simulink model "TST_EGRVlv_VDMon"  (R2016b)
settings: Solver=FixedStepDiscrete  StartTime=0.0  StopTime=simTime  FixedStep=sampleTime  RelTol=1e-3
values from neighbouring files (symbols this model uses):
  testCase = 1    [initTST_EGRVlv_VDMon_001.m]
libraries: UnitTest_Lib x6, simulink x2
settings Model: Creator=liangyunbo  LastModifiedBy=liangyunbo
settings DebuggingCC: SignalRangeChecking=error

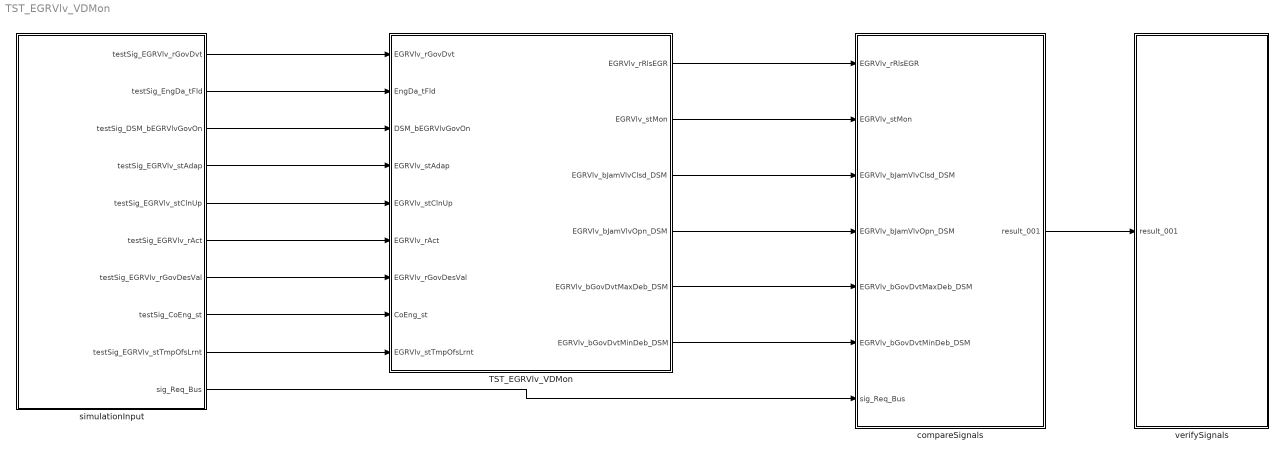
== system TST_EGRVlv_VDMon ==
  TST_EGRVlv_VDMon : Subsystem
  compareSignals : Subsystem
  simulationInput : Subsystem
  verifySignals : Subsystem
  wires:
  simulationInput/1(testSig_EGRVlv_rGovDvt) -> TST_EGRVlv_VDMon/1(EGRVlv_rGovDvt)
  simulationInput/2(testSig_EngDa_tFld) -> TST_EGRVlv_VDMon/2(EngDa_tFld)
  simulationInput/3(testSig_DSM_bEGRVlvGovOn) -> TST_EGRVlv_VDMon/3(DSM_bEGRVlvGovOn)
  simulationInput/4(testSig_EGRVlv_stAdap) -> TST_EGRVlv_VDMon/4(EGRVlv_stAdap)
  simulationInput/5(testSig_EGRVlv_stClnUp) -> TST_EGRVlv_VDMon/5(EGRVlv_stClnUp)
  simulationInput/6(testSig_EGRVlv_rAct) -> TST_EGRVlv_VDMon/6(EGRVlv_rAct)
  simulationInput/7(testSig_EGRVlv_rGovDesVal) -> TST_EGRVlv_VDMon/7(EGRVlv_rGovDesVal)
  simulationInput/8(testSig_CoEng_st) -> TST_EGRVlv_VDMon/8(CoEng_st)
  simulationInput/9(testSig_EGRVlv_stTmpOfsLrnt) -> TST_EGRVlv_VDMon/9(EGRVlv_stTmpOfsLrnt)
  TST_EGRVlv_VDMon/1(EGRVlv_rRlsEGR) -> compareSignals/1(EGRVlv_rRlsEGR)
  TST_EGRVlv_VDMon/2(EGRVlv_stMon) -> compareSignals/2(EGRVlv_stMon)
  TST_EGRVlv_VDMon/3(EGRVlv_bJamVlvClsd_DSM) -> compareSignals/3(EGRVlv_bJamVlvClsd_DSM)
  TST_EGRVlv_VDMon/4(EGRVlv_bJamVlvOpn_DSM) -> compareSignals/4(EGRVlv_bJamVlvOpn_DSM)
  TST_EGRVlv_VDMon/5(EGRVlv_bGovDvtMaxDeb_DSM) -> compareSignals/5(EGRVlv_bGovDvtMaxDeb_DSM)
  TST_EGRVlv_VDMon/6(EGRVlv_bGovDvtMinDeb_DSM) -> compareSignals/6(EGRVlv_bGovDvtMinDeb_DSM)
  simulationInput/10(sig_Req_Bus) -> compareSignals/7(sig_Req_Bus)
  compareSignals/1(result_001) -> verifySignals/1(result_001)

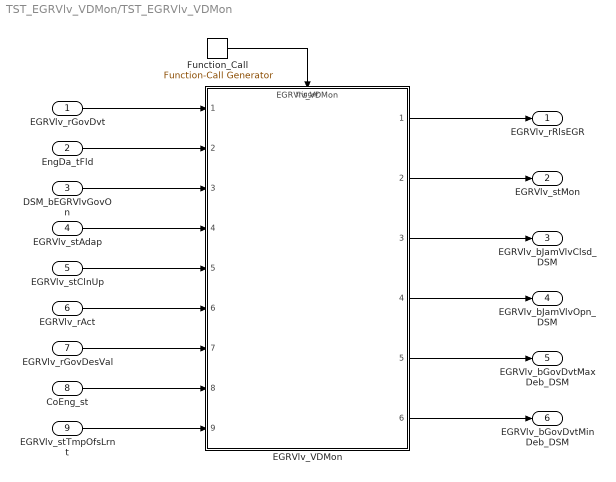
== system TST_EGRVlv_VDMon/TST_EGRVlv_VDMon ==
  EGRVlv_rGovDvt : Inport
  EngDa_tFld : Inport  Port=2
  DSM_bEGRVlvGovOn : Inport  Port=3
  EGRVlv_stAdap : Inport  Port=4
  EGRVlv_stClnUp : Inport  Port=5
  EGRVlv_rAct : Inport  Port=6
  EGRVlv_rGovDesVal : Inport  Port=7
  CoEng_st : Inport  Port=8
  EGRVlv_stTmpOfsLrnt : Inport  Port=9
  EGRVlv_VDMon : ModelReference  ModelNameDialog=EGRVlv_VDMon  SimulationMode=Normal  ModelReferenceVersion=1.16  TriggerPortName=function  TriggerPortTriggerType=function-call  TriggerPortStatesWhenEnabling=held
  Function_Call : simulink/Ports & Subsystems/Function-Call Generator  sample_time=sampleTime  numberOfIterations=1
  EGRVlv_rRlsEGR : Outport
  EGRVlv_stMon : Outport  Port=2
  EGRVlv_bJamVlvClsd_DSM : Outport  Port=3
  EGRVlv_bJamVlvOpn_DSM : Outport  Port=4
  EGRVlv_bGovDvtMaxDeb_DSM : Outport  Port=5
  EGRVlv_bGovDvtMinDeb_DSM : Outport  Port=6
  wires:
  Function_Call/1 -> EGRVlv_VDMon/Trigger
  EGRVlv_rGovDvt/1 -> EGRVlv_VDMon/1
  EngDa_tFld/1 -> EGRVlv_VDMon/2
  DSM_bEGRVlvGovOn/1 -> EGRVlv_VDMon/3
  EGRVlv_stAdap/1 -> EGRVlv_VDMon/4
  EGRVlv_stClnUp/1 -> EGRVlv_VDMon/5
  EGRVlv_rAct/1 -> EGRVlv_VDMon/6
  EGRVlv_rGovDesVal/1 -> EGRVlv_VDMon/7
  CoEng_st/1 -> EGRVlv_VDMon/8
  EGRVlv_stTmpOfsLrnt/1 -> EGRVlv_VDMon/9
  EGRVlv_VDMon/1 -> EGRVlv_rRlsEGR/1
  EGRVlv_VDMon/2 -> EGRVlv_stMon/1
  EGRVlv_VDMon/3 -> EGRVlv_bJamVlvClsd_DSM/1
  EGRVlv_VDMon/4 -> EGRVlv_bJamVlvOpn_DSM/1
  EGRVlv_VDMon/5 -> EGRVlv_bGovDvtMaxDeb_DSM/1
  EGRVlv_VDMon/6 -> EGRVlv_bGovDvtMinDeb_DSM/1

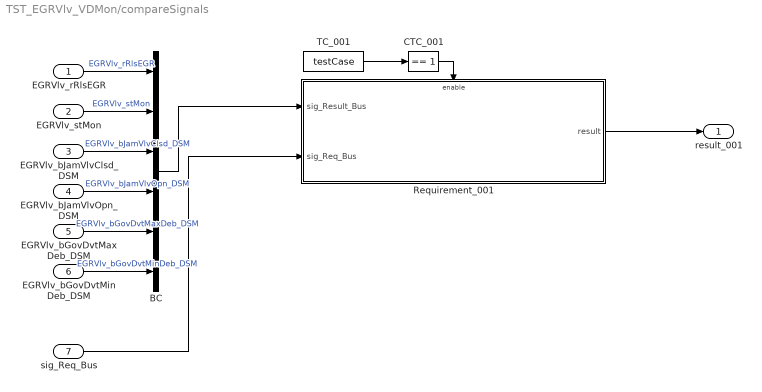
== system TST_EGRVlv_VDMon/compareSignals ==
  EGRVlv_rRlsEGR : Inport
  EGRVlv_stMon : Inport  Port=2
  EGRVlv_bJamVlvClsd_DSM : Inport  Port=3
  EGRVlv_bJamVlvOpn_DSM : Inport  Port=4
  EGRVlv_bGovDvtMaxDeb_DSM : Inport  Port=5
  EGRVlv_bGovDvtMinDeb_DSM : Inport  Port=6
  sig_Req_Bus : Inport  Port=7
  BC : BusCreator  Inputs=6
  CTC_001 : simulink/Logic and Bit Operations/Compare To Constant  relop===  const=1  OutDataTypeStr=boolean
  Requirement_001 : Subsystem
  TC_001 : Constant  Value=testCase
  result_001 : Outport
  wires:
  EGRVlv_rRlsEGR/1 -> BC/1  "EGRVlv_rRlsEGR"
  EGRVlv_stMon/1 -> BC/2  "EGRVlv_stMon"
  EGRVlv_bJamVlvClsd_DSM/1 -> BC/3  "EGRVlv_bJamVlvClsd_DSM"
  EGRVlv_bJamVlvOpn_DSM/1 -> BC/4  "EGRVlv_bJamVlvOpn_DSM"
  EGRVlv_bGovDvtMaxDeb_DSM/1 -> BC/5  "EGRVlv_bGovDvtMaxDeb_DSM"
  EGRVlv_bGovDvtMinDeb_DSM/1 -> BC/6  "EGRVlv_bGovDvtMinDeb_DSM"
  TC_001/1 -> CTC_001/1
  CTC_001/1 -> Requirement_001/Enable
  sig_Req_Bus/1 -> Requirement_001/2(sig_Req_Bus)
  BC/1 -> Requirement_001/1(sig_Result_Bus)
  Requirement_001/1(result) -> result_001/1

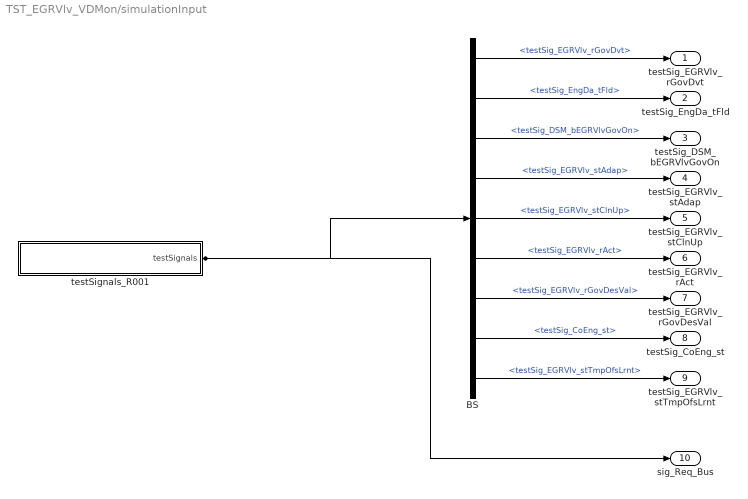
== system TST_EGRVlv_VDMon/simulationInput ==
  BS : BusSelector  OutputSignals=testSig_EGRVlv_rGovDvt,testSig_EngDa_tFld,testSig_DSM_bEGRVlvGovOn,testSig_EGRVlv_stAdap,testSig_EGRVlv_stClnUp,testSig_EGRVlv_rAct,testSig_EGRVlv_rGovDesVal,testSig_CoEng_st,testSig_EGRVlv_stTmpOfsLrnt
  testSignals_R001 : Subsystem
  testSig_EGRVlv_rGovDvt : Outport
  testSig_EngDa_tFld : Outport  Port=2
  testSig_DSM_bEGRVlvGovOn : Outport  Port=3
  testSig_EGRVlv_stAdap : Outport  Port=4
  testSig_EGRVlv_stClnUp : Outport  Port=5
  testSig_EGRVlv_rAct : Outport  Port=6
  testSig_EGRVlv_rGovDesVal : Outport  Port=7
  testSig_CoEng_st : Outport  Port=8
  testSig_EGRVlv_stTmpOfsLrnt : Outport  Port=9
  sig_Req_Bus : Outport  Port=10
  wires:
  BS/1 -> testSig_EGRVlv_rGovDvt/1  "<testSig_EGRVlv_rGovDvt>"
  BS/2 -> testSig_EngDa_tFld/1  "<testSig_EngDa_tFld>"
  BS/3 -> testSig_DSM_bEGRVlvGovOn/1  "<testSig_DSM_bEGRVlvGovOn>"
  BS/4 -> testSig_EGRVlv_stAdap/1  "<testSig_EGRVlv_stAdap>"
  BS/5 -> testSig_EGRVlv_stClnUp/1  "<testSig_EGRVlv_stClnUp>"
  BS/6 -> testSig_EGRVlv_rAct/1  "<testSig_EGRVlv_rAct>"
  BS/7 -> testSig_EGRVlv_rGovDesVal/1  "<testSig_EGRVlv_rGovDesVal>"
  BS/8 -> testSig_CoEng_st/1  "<testSig_CoEng_st>"
  BS/9 -> testSig_EGRVlv_stTmpOfsLrnt/1  "<testSig_EGRVlv_stTmpOfsLrnt>"
  testSignals_R001/1(testSignals) -> BS/1, sig_Req_Bus/1

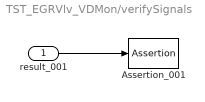
== system TST_EGRVlv_VDMon/verifySignals ==
  result_001 : Inport
  Assertion_001 : Assertion  Enabled=off
  wires:
  result_001/1 -> Assertion_001/1

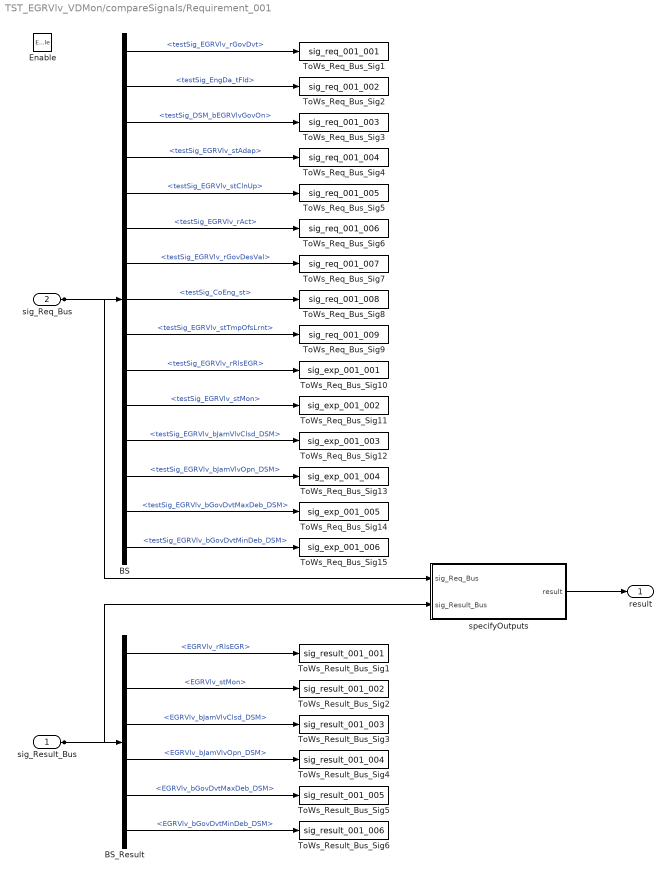
== system TST_EGRVlv_VDMon/compareSignals/Requirement_001 ==
  sig_Result_Bus : Inport
  sig_Req_Bus : Inport  Port=2
  Enable : EnablePort
  BS : BusSelector  OutputSignals=testSig_EGRVlv_rGovDvt,testSig_EngDa_tFld,testSig_DSM_bEGRVlvGovOn,testSig_EGRVlv_stAdap,testSig_EGRVlv_stClnUp,testSig_EGRVlv_rAct,testSig_EGRVlv_rGovDesVal,testSig_CoEng_st,testSig_EGRVlv_stTmpOfsLrnt,testSig_EGRVlv_rRlsEGR,testSig_EGRVlv_stMon,testSig_EGRVlv_bJamVlvClsd_DSM,testSig_EGRVlv_bJamVlvOpn_DSM,testSig_EGRVlv_bGovDvtMaxDeb_DSM,testSig_EGRVlv_bGovDvtMinDeb_DSM
  BS_Result : BusSelector  OutputSignals=EGRVlv_rRlsEGR,EGRVlv_stMon,EGRVlv_bJamVlvClsd_DSM,EGRVlv_bJamVlvOpn_DSM,EGRVlv_bGovDvtMaxDeb_DSM,EGRVlv_bGovDvtMinDeb_DSM
  ToWs_Req_Bus_Sig1 : ToWorkspace  VariableName=sig_req_001_001  SaveFormat=Structure With Time
  ToWs_Req_Bus_Sig10 : ToWorkspace  VariableName=sig_exp_001_001  SaveFormat=Structure With Time
  ToWs_Req_Bus_Sig11 : ToWorkspace  VariableName=sig_exp_001_002  SaveFormat=Structure With Time
  ToWs_Req_Bus_Sig12 : ToWorkspace  VariableName=sig_exp_001_003  SaveFormat=Structure With Time
  ToWs_Req_Bus_Sig13 : ToWorkspace  VariableName=sig_exp_001_004  SaveFormat=Structure With Time
  ToWs_Req_Bus_Sig14 : ToWorkspace  VariableName=sig_exp_001_005  SaveFormat=Structure With Time
  ToWs_Req_Bus_Sig15 : ToWorkspace  VariableName=sig_exp_001_006  SaveFormat=Structure With Time
  ToWs_Req_Bus_Sig2 : ToWorkspace  VariableName=sig_req_001_002  SaveFormat=Structure With Time
  ToWs_Req_Bus_Sig3 : ToWorkspace  VariableName=sig_req_001_003  SaveFormat=Structure With Time
  ToWs_Req_Bus_Sig4 : ToWorkspace  VariableName=sig_req_001_004  SaveFormat=Structure With Time
  ToWs_Req_Bus_Sig5 : ToWorkspace  VariableName=sig_req_001_005  SaveFormat=Structure With Time
  ToWs_Req_Bus_Sig6 : ToWorkspace  VariableName=sig_req_001_006  SaveFormat=Structure With Time
  ToWs_Req_Bus_Sig7 : ToWorkspace  VariableName=sig_req_001_007  SaveFormat=Structure With Time
  ToWs_Req_Bus_Sig8 : ToWorkspace  VariableName=sig_req_001_008  SaveFormat=Structure With Time
  ToWs_Req_Bus_Sig9 : ToWorkspace  VariableName=sig_req_001_009  SaveFormat=Structure With Time
  ToWs_Result_Bus_Sig1 : ToWorkspace  VariableName=sig_result_001_001  SaveFormat=Structure With Time
  ToWs_Result_Bus_Sig2 : ToWorkspace  VariableName=sig_result_001_002  SaveFormat=Structure With Time
  ToWs_Result_Bus_Sig3 : ToWorkspace  VariableName=sig_result_001_003  SaveFormat=Structure With Time
  ToWs_Result_Bus_Sig4 : ToWorkspace  VariableName=sig_result_001_004  SaveFormat=Structure With Time
  ToWs_Result_Bus_Sig5 : ToWorkspace  VariableName=sig_result_001_005  SaveFormat=Structure With Time
  ToWs_Result_Bus_Sig6 : ToWorkspace  VariableName=sig_result_001_006  SaveFormat=Structure With Time
  specifyOutputs : Subsystem
  result : Outport
  wires:
  sig_Req_Bus/1 -> BS/1, specifyOutputs/1(sig_Req_Bus)
  BS/1 -> ToWs_Req_Bus_Sig1/1  "<testSig_EGRVlv_rGovDvt>"
  BS/2 -> ToWs_Req_Bus_Sig2/1  "<testSig_EngDa_tFld>"
  BS/3 -> ToWs_Req_Bus_Sig3/1  "<testSig_DSM_bEGRVlvGovOn>"
  BS/4 -> ToWs_Req_Bus_Sig4/1  "<testSig_EGRVlv_stAdap>"
  BS/5 -> ToWs_Req_Bus_Sig5/1  "<testSig_EGRVlv_stClnUp>"
  BS/6 -> ToWs_Req_Bus_Sig6/1  "<testSig_EGRVlv_rAct>"
  BS/7 -> ToWs_Req_Bus_Sig7/1  "<testSig_EGRVlv_rGovDesVal>"
  BS/8 -> ToWs_Req_Bus_Sig8/1  "<testSig_CoEng_st>"
  BS/9 -> ToWs_Req_Bus_Sig9/1  "<testSig_EGRVlv_stTmpOfsLrnt>"
  BS/10 -> ToWs_Req_Bus_Sig10/1  "<testSig_EGRVlv_rRlsEGR>"
  BS/11 -> ToWs_Req_Bus_Sig11/1  "<testSig_EGRVlv_stMon>"
  BS/12 -> ToWs_Req_Bus_Sig12/1  "<testSig_EGRVlv_bJamVlvClsd_DSM>"
  BS/13 -> ToWs_Req_Bus_Sig13/1  "<testSig_EGRVlv_bJamVlvOpn_DSM>"
  BS/14 -> ToWs_Req_Bus_Sig14/1  "<testSig_EGRVlv_bGovDvtMaxDeb_DSM>"
  BS/15 -> ToWs_Req_Bus_Sig15/1  "<testSig_EGRVlv_bGovDvtMinDeb_DSM>"
  sig_Result_Bus/1 -> BS_Result/1, specifyOutputs/2(sig_Result_Bus)
  BS_Result/1 -> ToWs_Result_Bus_Sig1/1  "<EGRVlv_rRlsEGR>"
  BS_Result/2 -> ToWs_Result_Bus_Sig2/1  "<EGRVlv_stMon>"
  BS_Result/3 -> ToWs_Result_Bus_Sig3/1  "<EGRVlv_bJamVlvClsd_DSM>"
  BS_Result/4 -> ToWs_Result_Bus_Sig4/1  "<EGRVlv_bJamVlvOpn_DSM>"
  BS_Result/5 -> ToWs_Result_Bus_Sig5/1  "<EGRVlv_bGovDvtMaxDeb_DSM>"
  BS_Result/6 -> ToWs_Result_Bus_Sig6/1  "<EGRVlv_bGovDvtMinDeb_DSM>"
  specifyOutputs/1(result) -> result/1

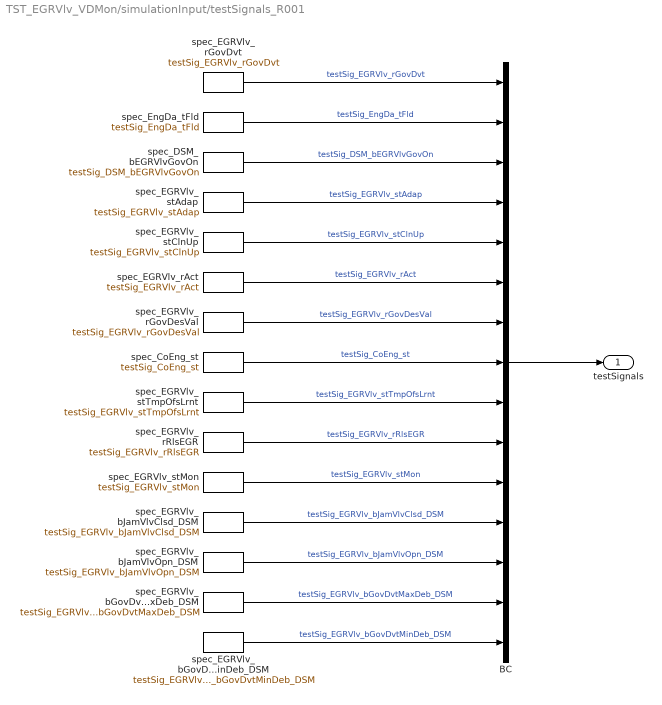
== system TST_EGRVlv_VDMon/simulationInput/testSignals_R001 ==
  BC : BusCreator  Inputs=15
  spec_CoEng_st : FromWorkspace  VariableName=testSig_CoEng_st  Interpolate=off  OutputAfterFinalValue=Holding final value
  spec_DSM_bEGRVlvGovOn : FromWorkspace  VariableName=testSig_DSM_bEGRVlvGovOn  Interpolate=off  OutputAfterFinalValue=Holding final value
  spec_EGRVlv_bGovDvtMaxDeb_DSM : FromWorkspace  VariableName=testSig_EGRVlv_bGovDvtMaxDeb_DSM  Interpolate=off  OutputAfterFinalValue=Holding final value
  spec_EGRVlv_bGovDvtMinDeb_DSM : FromWorkspace  VariableName=testSig_EGRVlv_bGovDvtMinDeb_DSM  Interpolate=off  OutputAfterFinalValue=Holding final value
  spec_EGRVlv_bJamVlvClsd_DSM : FromWorkspace  VariableName=testSig_EGRVlv_bJamVlvClsd_DSM  Interpolate=off  OutputAfterFinalValue=Holding final value
  spec_EGRVlv_bJamVlvOpn_DSM : FromWorkspace  VariableName=testSig_EGRVlv_bJamVlvOpn_DSM  Interpolate=off  OutputAfterFinalValue=Holding final value
  spec_EGRVlv_rAct : FromWorkspace  VariableName=testSig_EGRVlv_rAct  Interpolate=off  OutputAfterFinalValue=Holding final value
  spec_EGRVlv_rGovDesVal : FromWorkspace  VariableName=testSig_EGRVlv_rGovDesVal  Interpolate=off  OutputAfterFinalValue=Holding final value
  spec_EGRVlv_rGovDvt : FromWorkspace  VariableName=testSig_EGRVlv_rGovDvt  Interpolate=off  OutputAfterFinalValue=Holding final value
  spec_EGRVlv_rRlsEGR : FromWorkspace  VariableName=testSig_EGRVlv_rRlsEGR  Interpolate=off  OutputAfterFinalValue=Holding final value
  spec_EGRVlv_stAdap : FromWorkspace  VariableName=testSig_EGRVlv_stAdap  Interpolate=off  OutputAfterFinalValue=Holding final value
  spec_EGRVlv_stClnUp : FromWorkspace  VariableName=testSig_EGRVlv_stClnUp  Interpolate=off  OutputAfterFinalValue=Holding final value
  spec_EGRVlv_stMon : FromWorkspace  VariableName=testSig_EGRVlv_stMon  Interpolate=off  OutputAfterFinalValue=Holding final value
  spec_EGRVlv_stTmpOfsLrnt : FromWorkspace  VariableName=testSig_EGRVlv_stTmpOfsLrnt  Interpolate=off  OutputAfterFinalValue=Holding final value
  spec_EngDa_tFld : FromWorkspace  VariableName=testSig_EngDa_tFld  Interpolate=off  OutputAfterFinalValue=Holding final value
  testSignals : Outport
  wires:
  BC/1 -> testSignals/1
  spec_EGRVlv_rGovDvt/1 -> BC/1  "testSig_EGRVlv_rGovDvt"
  spec_EngDa_tFld/1 -> BC/2  "testSig_EngDa_tFld"
  spec_DSM_bEGRVlvGovOn/1 -> BC/3  "testSig_DSM_bEGRVlvGovOn"
  spec_EGRVlv_stAdap/1 -> BC/4  "testSig_EGRVlv_stAdap"
  spec_EGRVlv_stClnUp/1 -> BC/5  "testSig_EGRVlv_stClnUp"
  spec_EGRVlv_rAct/1 -> BC/6  "testSig_EGRVlv_rAct"
  spec_EGRVlv_rGovDesVal/1 -> BC/7  "testSig_EGRVlv_rGovDesVal"
  spec_CoEng_st/1 -> BC/8  "testSig_CoEng_st"
  spec_EGRVlv_stTmpOfsLrnt/1 -> BC/9  "testSig_EGRVlv_stTmpOfsLrnt"
  spec_EGRVlv_rRlsEGR/1 -> BC/10  "testSig_EGRVlv_rRlsEGR"
  spec_EGRVlv_stMon/1 -> BC/11  "testSig_EGRVlv_stMon"
  spec_EGRVlv_bJamVlvClsd_DSM/1 -> BC/12  "testSig_EGRVlv_bJamVlvClsd_DSM"
  spec_EGRVlv_bJamVlvOpn_DSM/1 -> BC/13  "testSig_EGRVlv_bJamVlvOpn_DSM"
  spec_EGRVlv_bGovDvtMaxDeb_DSM/1 -> BC/14  "testSig_EGRVlv_bGovDvtMaxDeb_DSM"
  spec_EGRVlv_bGovDvtMinDeb_DSM/1 -> BC/15  "testSig_EGRVlv_bGovDvtMinDeb_DSM"

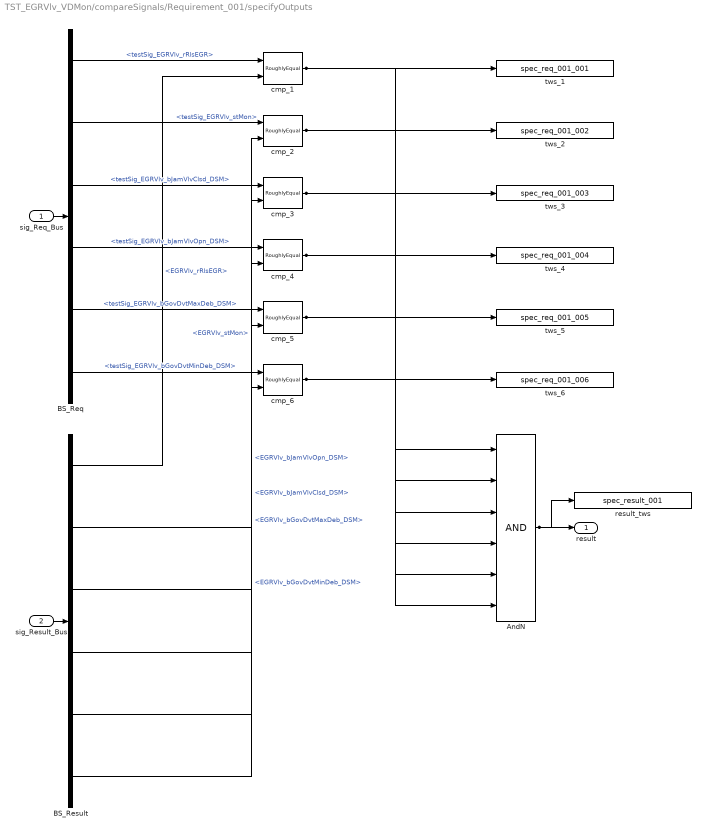
== system TST_EGRVlv_VDMon/compareSignals/Requirement_001/specifyOutputs ==
  sig_Req_Bus : Inport
  sig_Result_Bus : Inport  Port=2
  AndN : Logic  Inputs=6
  BS_Req : BusSelector  OutputSignals=testSig_EGRVlv_rRlsEGR,testSig_EGRVlv_stMon,testSig_EGRVlv_bJamVlvClsd_DSM,testSig_EGRVlv_bJamVlvOpn_DSM,testSig_EGRVlv_bGovDvtMaxDeb_DSM,testSig_EGRVlv_bGovDvtMinDeb_DSM
  BS_Result : BusSelector  OutputSignals=EGRVlv_rRlsEGR,EGRVlv_stMon,EGRVlv_bJamVlvClsd_DSM,EGRVlv_bJamVlvOpn_DSM,EGRVlv_bGovDvtMaxDeb_DSM,EGRVlv_bGovDvtMinDeb_DSM
  cmp_{1..6} (6 alike) : UnitTest_Lib/RoughlyEqual  slope=0.1
  result_tws : ToWorkspace  VariableName=spec_result_001
  tws_1 : ToWorkspace  VariableName=spec_req_001_001
  tws_2 : ToWorkspace  VariableName=spec_req_001_002
  tws_3 : ToWorkspace  VariableName=spec_req_001_003
  tws_4 : ToWorkspace  VariableName=spec_req_001_004
  tws_5 : ToWorkspace  VariableName=spec_req_001_005
  tws_6 : ToWorkspace  VariableName=spec_req_001_006
  result : Outport
  wires:
  sig_Req_Bus/1 -> BS_Req/1
  sig_Result_Bus/1 -> BS_Result/1
  AndN/1 -> result/1, result_tws/1
  BS_Req/1 -> cmp_1/1  "<testSig_EGRVlv_rRlsEGR>"
  BS_Result/1 -> cmp_1/2  "<EGRVlv_rRlsEGR>"
  cmp_1/1 -> tws_1/1, AndN/1
  BS_Req/2 -> cmp_2/1  "<testSig_EGRVlv_stMon>"
  BS_Result/2 -> cmp_2/2  "<EGRVlv_stMon>"
  cmp_2/1 -> tws_2/1, AndN/2
  BS_Req/3 -> cmp_3/1  "<testSig_EGRVlv_bJamVlvClsd_DSM>"
  BS_Result/3 -> cmp_3/2  "<EGRVlv_bJamVlvClsd_DSM>"
  cmp_3/1 -> tws_3/1, AndN/3
  BS_Req/4 -> cmp_4/1  "<testSig_EGRVlv_bJamVlvOpn_DSM>"
  BS_Result/4 -> cmp_4/2  "<EGRVlv_bJamVlvOpn_DSM>"
  cmp_4/1 -> tws_4/1, AndN/4
  BS_Req/5 -> cmp_5/1  "<testSig_EGRVlv_bGovDvtMaxDeb_DSM>"
  BS_Result/5 -> cmp_5/2  "<EGRVlv_bGovDvtMaxDeb_DSM>"
  cmp_5/1 -> tws_5/1, AndN/5
  BS_Req/6 -> cmp_6/1  "<testSig_EGRVlv_bGovDvtMinDeb_DSM>"
  BS_Result/6 -> cmp_6/2  "<EGRVlv_bGovDvtMinDeb_DSM>"
  cmp_6/1 -> tws_6/1, AndN/6
